simulink model "simu_png_radome_ukf_dgp"  (R2020a)
settings: Solver=ode4  StartTime=0.0  StopTime=20  FixedStep=0.001  RelTol=1e-3
values from neighbouring files (symbols this model uses):
  N = 4    [initial.m]
  T_alpha = 1    [initial.m]
  tau = 0.1    [initial.m]
  V_M = 500    [initial.m]
settings Model: Creator=admin  LastModifiedBy=admin

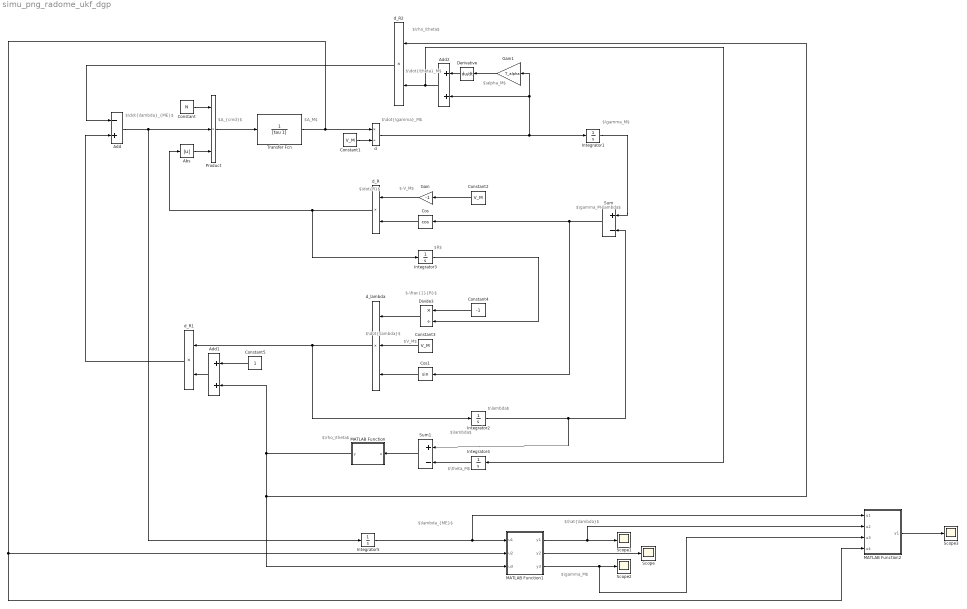
== system simu_png_radome_ukf_dgp ==
  note: $\dot{\lambda}$
  note: $\lambda$
  note: $\gamma_M$
  note: $-\frac{1}{R}$
  note: $V_M$
  note: $\gamma_M-\lambda$
  note: $-V_M$
  note: $\dot{R}$
  note: $A_{cmd}$
  note: $A_M$
  note: $\dot{\gamma}_M$
  note: $R$
  note: $\dot{\theta}_M$
  note: $\dot{\lambda}_{ME}$
  note: $\theta_M$
  note: $\lambda$
  note: $\rho_\theta$
  note: $\rho_\theta$
  note: $\alpha_M$
  note: $\lambda_{ME}$
  note: $\hat{\lambda}$
  note: $\gamma_M$
  Abs : Abs
  Add : Sum  Inputs=-+
  Add1 : Sum
  Add2 : Sum
  Constant : Constant  Value=N
  Constant1 : Constant  Value=V_M
  Constant2 : Constant  Value=V_M
  Constant3 : Constant  Value=V_M
  Constant4 : Constant  Value=-1
  Constant5 : Constant
  Cos : Trigonometry  Operator=cos
  Cos1 : Trigonometry
  Derivative : Derivative
  Divide3 : Product  Inputs=*/
  Gain : Gain  Gain=-1
  Gain1 : Gain  Gain=T_alpha
  Integrator1 : Integrator
  Integrator2 : Integrator  InitialCondition=0.0997
  Integrator3 : Integrator  InitialCondition=10050
  Integrator4 : Integrator
  Integrator5 : Integrator  InitialCondition=0.1021925
  MATLAB Function : MATLAB Function  TreatAsAtomicUnit=on
  MATLAB Function1 : MATLAB Function  TreatAsAtomicUnit=on
  MATLAB Function2 : MATLAB Function  TreatAsAtomicUnit=on
  Product : Product  Inputs=3
  Scope{,1..3} (4 alike) : Scope
  Sum : Sum  Inputs=+|-
  Sum1 : Sum  Inputs=+|-
  Transfer Fcn : TransferFcn  Denominator=[tau 1]
  d : Product  Inputs=*/
  d_R : Product  Inputs=**
  d_R1 : Product  Inputs=**
  d_R2 : Product  Inputs=**
  d_lambda : Product  Inputs=***
  wires:
  Transfer Fcn/1 -> d/1, MATLAB Function2/4(u4), MATLAB Function1/2(u2)
  Integrator3/1 -> Divide3/2
  Constant/1 -> Product/1
  Product/1 -> Transfer Fcn/1
  Abs/1 -> Product/3
  Constant1/1 -> d/2
  Gain/1 -> d_R/1
  Constant2/1 -> Gain/1
  Cos/1 -> d_R/2
  d_R/1 -> Integrator3/1, Abs/1
  Divide3/1 -> d_lambda/1
  Constant3/1 -> d_lambda/2
  Cos1/1 -> d_lambda/3
  Sum/1 -> Cos1/1, Cos/1
  Integrator1/1 -> Sum/1
  d_lambda/1 -> Integrator2/1, d_R1/1
  Constant4/1 -> Divide3/1
  d/1 -> Add2/2, Gain1/1, Integrator1/1
  Add/1 -> Integrator5/1, Product/2
  Add1/1 -> d_R1/2
  Constant5/1 -> Add1/1
  d_R1/1 -> Add/2
  Derivative/1 -> Add2/1
  Add2/1 -> d_R2/2, Integrator4/1
  d_R2/1 -> Add/1
  Integrator4/1 -> Sum1/2
  Sum1/1 -> MATLAB Function/1(u)
  MATLAB Function/1(y) -> Add1/2, MATLAB Function1/3(u3), d_R2/1
  Gain1/1 -> Derivative/1
  Integrator2/1 -> Sum1/1, Sum/2
  Integrator5/1 -> MATLAB Function2/1(u1), MATLAB Function1/1(u1)
  MATLAB Function1/2(y2) -> Scope/1
  MATLAB Function1/1(y1) -> MATLAB Function2/2(u2), Scope1/1
  MATLAB Function1/3(y3) -> Scope2/1, MATLAB Function2/3(u3)
  MATLAB Function2/1(y1) -> Scope3/1

== matlab function simu_png_radome_ukf_dgp/MATLAB Function1 ==
  settings: updateMethod=DISCRETE
  data: u1 input; y1 output; u2 input; u3 input; y2 output; y3 output
function [y1,y2,y3]=fcn(u1,u2,u3)



%% read data
z_curr=u1;
A_M_curr=u2;
rho_theta_curr=u3;% first assume that rho_theta is known as an input, while it is supposed to be provided by GPR

t_end=20;
delta_t_cont=0.001;
delta_t_disc=0.001;
T=t_end/delta_t_disc;

T_alpha=1;
V_M=500;

persistent i_curr
persistent u_cont
persistent x_est
persistent P_est
persistent rho_theta


if isempty(i_curr)
    i_curr=1;
else
    i_curr=i_curr+1;
end

if isempty(u_cont)
    u_cont=zeros(T+1,1);
    u_cont(1)=A_M_curr;
else
    u_cont(i_curr)=A_M_curr;
end

if isempty(rho_theta)
    rho_theta=zeros(T+1,1);
    rho_theta(1)=rho_theta_curr;
else
    rho_theta(i_curr)=rho_theta_curr;
end

%% (1) set covariance of process noise
Q_1=(deg2rad(1e-3))^2;
Q_2=5*1e2;
Q_3=(deg2rad(1e-3))^2;
Q_filter=diag([Q_1,Q_2,Q_3]);

%% (2) set covariance of measurement noise
R_filter=(deg2rad(5*1e-3))^2;

%% (2) initial
if isempty(x_est)
    x_est=zeros(T+1,3);
end
if isempty(P_est)
    P_est=zeros(T+1,3,3);
end
x_0=zeros(3,1);
x_0(1)=deg2rad(7.7106);
x_0(2)=12050;
x_0(3)=deg2rad(2);
P_0=zeros(3,3);
P_0(1,1)=(deg2rad(1))^2;
P_0(2,2)=(1e3)^2;
P_0(3,3)=(deg2rad(1))^2;

%% (3) main loop
if i_curr==1
    x_corr=x_0;
    P_corr=P_0;
else
    x_prev=(x_est(i_curr-1,:))';
    P_prev=shiftdim(P_est(i_curr-1,:,:));   
    [x_pred,P_pred,x_corr,P_corr]=function_ukf(x_prev,P_prev,z_curr,Q_filter,R_filter,delta_t_disc,delta_t_cont,rho_theta,T_alpha,V_M,u_cont,i_curr);

end
x_est(i_curr,:)=x_corr';
P_est(i_curr,:,:)=P_corr;
% y=[u1;u2;u3];
y1=x_corr(1);
y2=x_corr(2);
y3=x_corr(3);

== matlab function simu_png_radome_ukf_dgp/MATLAB Function ==
  data: u input; y output
function y = fcn(u)

%%
% r=-0.5;
% zeta=4;
% p=1;
% 
% if u<0
%     a=exp(zeta*u);
%     b=zeta*sin(2*pi*u/p);
%     c=2*pi/p*cos(2*pi*u/p);
% else
%     a=exp(-zeta*u);
%     b=-zeta*sin(2*pi*u/p);
%     c=2*pi/p*cos(2*pi*u/p);
% end
% 
% y=r*a*(b+c);
% y=y/rad2deg(1);

%%
y=0.025;
% y=0.05;

== matlab function simu_png_radome_ukf_dgp/MATLAB Function2 ==
  settings: updateMethod=DISCRETE
  data: u1 input; y1 output; u2 input; u3 input; u4 input
function y1 =fcn(u1,u2,u3,u4)

%% read data
lambda_ME_curr=u1;

lambda_curr=u2;
gamma_M_curr=u3;
A_M_curr=u4;



t_end=20;
delta_t_cont=0.001;
delta_t_disc=0.001;
T=t_end/delta_t_disc;

T_alpha=1;
V_M=500;

persistent i_curr
persistent theta_s_est
persistent lambda_r_est

if isempty(i_curr)
    i_curr=1;
else
    i_curr=i_curr+1;
end

if isempty(theta_s_est)
    theta_s_est=zeros(T+1,1);
end

if isempty(lambda_r_est)
    lambda_r_est=zeros(T+1,1);
end

%% calculate look angle (theta_s)
% calculate alpha_M
alpha_M_curr=T_alpha*A_M_curr/V_M;

% calculate theta_M
theta_M_curr=gamma_M_curr+alpha_M_curr;

% calculate theta_s
theta_s_curr=lambda_curr-theta_M_curr;
theta_s_est(i_curr)=theta_s_curr;

%% calculate radome error
lambda_r_curr=lambda_ME_curr-lambda_curr;
lambda_r_est(i_curr)=lambda_r_curr;

%% testing, plot radome error VS look angle
% if i_curr==5*1e3
%     figure
%     index_m_est=2/delta_t_disc:100:i_curr;
%     plot(rad2deg(theta_s_est(index_m_est)),rad2deg(lambda_r_est(index_m_est)))
% end


%% calculate radome slope via Gaussian process

if i_curr==T+1
    index_m_est=2/delta_t_disc:100:i_curr;
    Xm_est=rad2deg(theta_s_est(index_m_est));
    Xm_est=Xm_est';
    fmh_est=rad2deg(lambda_r_est(index_m_est));
    
    % tuning hyperparameters
    lf_est=1;
    lx_est=1;
    % sfm_est=0.1;
    sfm_est=0.5;
    % hyp=function_gp_hyperparam(Xm_est,fmh_est);
    % lx_est = sqrt(hyp(1));
    % lf_est = sqrt(hyp(2));
    % sfm_est = sqrt(hyp(3));

    index_s_est=2/delta_t_disc:75:i_curr;
    Xs_est=rad2deg(theta_s_est(index_s_est));
    Xs_est=Xs_est';
    
    % GPR
    [mPost_est,SPost_est,mdPost_est,SdPost_est]=function_gp_dgp(Xs_est,Xm_est,fmh_est,lf_est,lx_est,sfm_est);
    sPost_est=sqrt(diag(SPost_est)); % These are the posterior standard deviations.
    sdPost_est=sqrt(diag(SdPost_est)); % These are the posterior standard deviations of the derivative.
    
    % testing
    
    figure
    hold on;
    grid on;
    plot(Xs_est, mPost_est, 'b-', 'LineWidth', 1); % We plot the mean line.
    plot(Xm_est, fmh_est, 'ro'); % We plot the measurement points.
    title('radome error VS look angle (GPR estimate)')
    xlabel('\theta_s (deg)')
    ylabel('\lambda_r (deg)')
    axis square
    
    figure
    hold on;
    grid on;
    plot(Xs_est, mdPost_est, 'b-', 'LineWidth', 1); % We plot the mean line.
    title('radome slope VS look angle (GPR estimate)')
    xlabel('\theta_s (deg)')
    ylabel('\rho_theta (deg/deg)')
    axis square
    
end

%% output
y1=u1;
